simulink model "FonctionBF"  (R2020a)
settings: Solver=VariableStepAuto  StartTime=0.0  StopTime=0.04  RelTol=1e-3
values from neighbouring files (symbols this model uses):
  denC = [ti 0]    [correcteur.m]    (also in correcteur2.m)
  denCD = [Rmoteur*tm Rmoteur]    [correcteur.m]
  denCR = [t1*t2 t1+t2 1]    [correcteur.m]
  numC = [t 1]    [correcteur.m]    (also in correcteur2.m = [tm 1])
  numCD = [2*E]    [correcteur.m]
  numCR = [Kretour]    [correcteur.m]
settings Model: Creator=predon  LastModifiedBy=predon

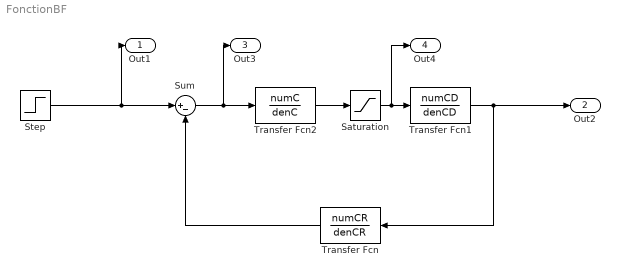
== system FonctionBF ==
  Saturation : Saturate
  Step : Step  Time=0.02  After=1.65  SampleTime=0
  Sum : Sum  Inputs=|+-
  Transfer Fcn : TransferFcn  Numerator=numCR  Denominator=denCR
  Transfer Fcn1 : TransferFcn  Numerator=numCD  Denominator=denCD
  Transfer Fcn2 : TransferFcn  Numerator=numC  Denominator=denC
  Out1 : Outport  SignalName=Icons
  Out2 : Outport  Port=2  SignalName=Is
  Out3 : Outport  Port=3  SignalName=Erreur
  Out4 : Outport  Port=4  SignalName=Alpha
  wires:
  Transfer Fcn1/1 -> Out2/1, Transfer Fcn/1
  Step/1 -> Out1/1, Sum/1
  Sum/1 -> Out3/1, Transfer Fcn2/1
  Transfer Fcn/1 -> Sum/2
  Transfer Fcn2/1 -> Saturation/1
  Saturation/1 -> Out4/1, Transfer Fcn1/1
